simulink model "feedback_loop_2"  (Simulink 7.9)
settings: Solver=ode45  StartTime=0.0  StopTime=2000  RelTol=1e-3
settings Model: Creator=kr2112  LastModifiedBy=kr2112

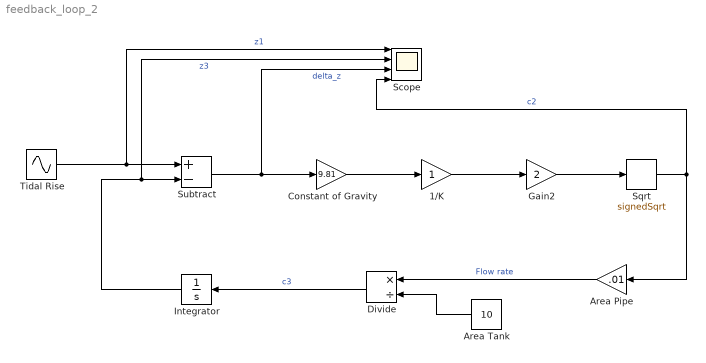
== system feedback_loop_2 ==
  1/K : Gain
  Area Pipe : Gain  Gain=.01
  Area Tank : Constant  Value=10
  Constant of Gravity : Gain  Gain=9.81
  Divide : Product  Inputs=*/
  Gain2 : Gain  Gain=2
  Integrator : Integrator
  Scope : Scope  NumInputPorts=4
      settings: YMin=-5~-5~-5~-5  YMax=5~5~5~5
  Sqrt : Sqrt  Operator=signedSqrt  SaturateOnIntegerOverflow=on
  Subtract : Sum  Inputs=+-
  Tidal Rise : Sin  Frequency=0.0083  SampleTime=0
  wires:
  Constant of Gravity/1 -> 1/K/1
  Sqrt/1 -> Scope/4, Area Pipe/1  "c2"
  Subtract/1 -> Constant of Gravity/1, Scope/3  "delta_z"
  Tidal Rise/1 -> Subtract/1, Scope/1  "z1"
  Integrator/1 -> Subtract/2, Scope/2  "z3"
  Gain2/1 -> Sqrt/1
  Area Pipe/1 -> Divide/1  "Flow rate"
  Area Tank/1 -> Divide/2
  Divide/1 -> Integrator/1  "c3"
  1/K/1 -> Gain2/1
